simulink model "classpractise"  (R2017b)
settings: Solver=VariableStepAuto  StartTime=0.0  StopTime=10.0  RelTol=1e-3
values from neighbouring files (symbols this model uses):
  g = 9.81    [mode.m]
undefined symbols (not defined in the file or in its folder): br, Km, Kv, L0, m
settings Model: Creator=Usuario  LastModifiedBy=Usuario

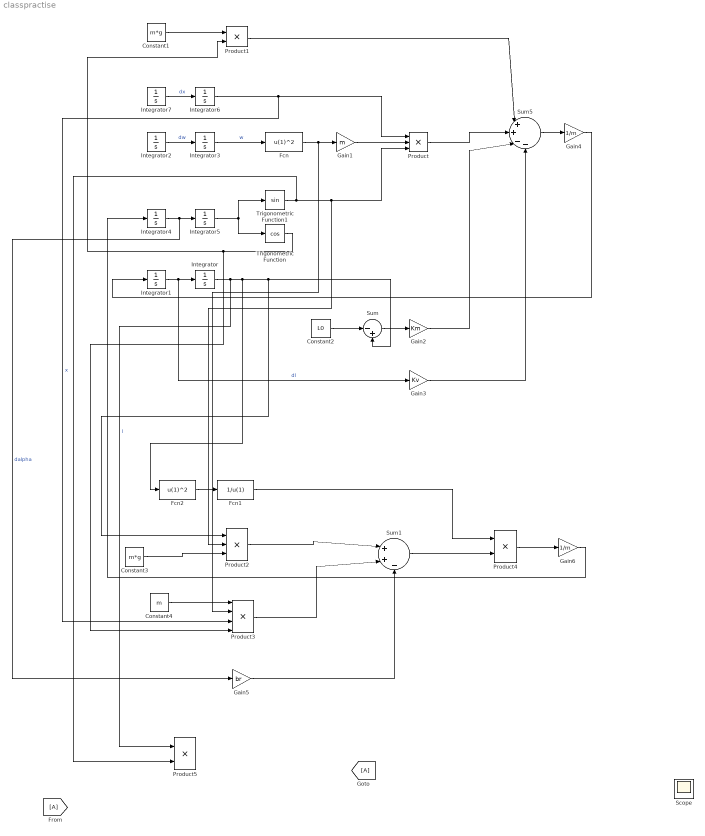
== system classpractise ==
  Constant1 : Constant  Value=m*g
  Constant2 : Constant  Value=L0
  Constant3 : Constant  Value=m*g
  Constant4 : Constant  Value=m
  Fcn : Fcn  Expr=u(1)^2
  Fcn1 : Fcn  Expr=1/u(1)
  Fcn2 : Fcn  Expr=u(1)^2
  Gain1 : Gain  Gain=m
  Gain2 : Gain  Gain=Km
  Gain3 : Gain  Gain=Kv
  Gain4 : Gain  Gain=1/m
  Gain5 : Gain  Gain=br
  Gain6 : Gain  Gain=1/m
  Integrator{,1..7} (8 alike) : Integrator
  Product : Product  Inputs=3
  Product1 : Product
  Product2 : Product  Inputs=3
  Product3 : Product  Inputs=4
  Product4 : Product
  Product5 : Product
  Scope : Scope
  Sum : Sum  Inputs=|-+
  Sum1 : Sum  Inputs=|++-
  Sum5 : Sum  Inputs=|++--
  Trigonometric Function : Trigonometry  Operator=cos
  Trigonometric Function1 : Trigonometry
  wires:
  Integrator1/1 -> Gain3/1, Integrator/1  "dl"
  Integrator/1 -> Fcn2/1, Sum/2, Product2/1, Product5/1  "l"
  Constant2/1 -> Sum/1
  Sum/1 -> Gain2/1
  Integrator4/1 -> Gain5/1, Integrator5/1  "dalpha"
  Integrator2/1 -> Integrator3/1  "dw"
  Integrator3/1 -> Fcn/1  "w"
  Fcn/1 -> Product3/2, Gain1/1
  Integrator7/1 -> Integrator6/1  "dx"
  Integrator5/1 -> Trigonometric Function1/1, Trigonometric Function/1
  Trigonometric Function1/1 -> Product5/2, Product2/2, Product/3
  Gain1/1 -> Product/2
  Integrator6/1 -> Product3/3, Product/1  "x"
  Constant1/1 -> Product1/1
  Trigonometric Function/1 -> Product3/4, Product1/2
  Product1/1 -> Sum5/1
  Product/1 -> Sum5/2
  Gain2/1 -> Sum5/3
  Gain3/1 -> Sum5/4
  Sum5/1 -> Gain4/1
  Gain4/1 -> Integrator1/1
  Fcn2/1 -> Fcn1/1
  Constant3/1 -> Product2/3
  Constant4/1 -> Product3/1
  Product2/1 -> Sum1/1
  Product3/1 -> Sum1/2
  Gain5/1 -> Sum1/3
  Sum1/1 -> Product4/2
  Fcn1/1 -> Product4/1
  Product4/1 -> Gain6/1
  Gain6/1 -> Integrator4/1
